simulink model "indexBase"  (Simulink 7.7)
settings: Solver=FixedStepDiscrete  StartTime=0.0  StopTime=10.0  FixedStep=1  RelTol=1e-3
settings Model: Creator=hnine  LastModifiedBy=hnine

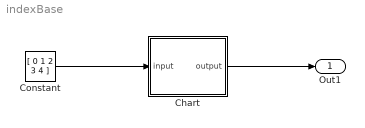
== system indexBase ==
  Chart : Stateflow chart  TreatAsAtomicUnit=on
  Constant : Constant  Value=[ 0 1 2 3 4 ]
  Out1 : Outport
  wires:
  Constant/1 -> Chart/1(input)
  Chart/1(output) -> Out1/1

== stateflow chart Chart ==
  (default) -> (junction 3) : { addend++; itr = 0;}
  (junction 3) -> (junction 4) [order 2]
  (junction 3) -> (junction 3) [order 1] : [itr <= 4 ]{ output[ itr + 3 ] = input[ itr + 2 ] + addend; itr++; }
  data: input input double size=5; output output double size=5; addend local double =0; itr local double =0
